simulink library "BrickPiSimSubLib_initreset"  (R2019a)
settings: Solver=VariableStepAuto  StartTime=0.0  StopTime=10.0  RelTol=1e-3
undefined symbols (not defined in the file or in its folder): A
libraries: BrickPiSimSubLib_Read x12, simulink x6, raspberrypilib x6
settings Model: Creator=hahn  LastModifiedBy=uk008555

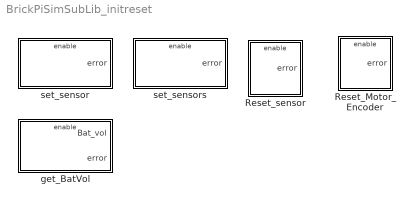
== system BrickPiSimSubLib_initreset ==
  Reset_Motor_Encoder : Subsystem  mask{Port_Val=A}
      mask prompts: Port_Val "Port"
      mask init:
      | switch Port_Val
      |     case 1
      |         d='A';
      |     case 2
      |         d='B';
      |     case 3
      |         d='C';
      |     otherwise
      |         d='D';
      | end
      mask TypeOptions Port_Val: Port_M/Port_Val
      mask Display: disp(['Reset\n Encoder \n Motor: ' d])
  Reset_sensor : Subsystem  mask{Port1_Val=on, Port2_Val=on, Port3_Val=on, Port4_Val=on}
      mask prompts: Port1_Val "Port1"; Port2_Val "Port2"; Port3_Val "Port3"; Port4_Val "Port4"
      mask init:
      | % d='';
      | % if Port1_Val
      | %     d=[d 'Sensor 1\n'];
      | % end
      | % if Port2_Val
      | %     d=[d 'Sensor 2\n'];
      | % end
      | % if Port3_Val
      | %     d=[d 'Sensor 3\n'];
      | % end
      | % if Port4_Val
      | %     d=[d 'Sensor 4'];
      | % end
      mask TypeOptions Port1_Val: Sensor_Ports/Port1_Val
      mask TypeOptions Port2_Val: Sensor_Ports/Port2_Val
      mask TypeOptions Port3_Val: Sensor_Ports/Port3_Val
      mask TypeOptions Port4_Val: Sensor_Ports/Port4_Val
      mask Display:
      | % disp(d)
      | [~,idx]=find([Port1_Val Port2_Val Port3_Val Port4_Val]);
      | disp(['Reset\n Sensor\n' num2str(idx)])
  get_BatVol : Subsystem
      mask Display: disp('Get\n VOLTAGE_BAT')
  set_sensor : Subsystem  mask{Type_Val=NXT Light on, Port_Val=3}
      mask prompts: Type_Val "Sensor Type:"; Port_Val "Port"
      mask init:
      | names = {
      |                   'NONE'
      |                   'I2C'
      |                   'CUSTOM'  % Choose 9v pullup, pin 5 and 6 configuration, and what to read back (ADC 1 and/or ADC 6 (always reports digital 5 and 6)).
      | 
      |                   'TOUCH'   % Touch sensor. When this mode is selected, automatically configure for NXT/EV3 as necessary.
      |                   'TOUCH_NXT' % 5
      |                   'TOUCH_EV3'
      | 
      |                   'NXT_LIGHT_ON'
      |                   'NXT_LIGHT_OFF'
      | 
      |                   'NXT_COLOR_RED'
      |                   'NXT_COLOR_GREEN'     % 10
      |                   'NXT_COLOR_BLUE'
      |                   'NXT_COLOR_FULL'
      |                   'NXT_COLOR_OFF'
      | 
      |                   'NXT_ULTRASONIC'
      | 
      |                   'EV3_GYRO_ABS'        % 15
      |                   'EV3_GYRO_DPS'
      |                   'EV3_GYRO_ABS_DPS'
      | 
      |                   'EV3_COLOR_REFLECTED'
      |                   'EV3_COLOR_AMBIENT'
      |                   'EV3_COLOR_COLOR'     % 20
      |                   'EV3_COLOR_RAW_REFLECTED'
      |                   'EV3_COLOR_COLOR_COMPONENTS'
      | 
      |                   'EV3_ULTRASONIC_CM'
      |                   'EV3_ULTRASONIC_INCHES'
      |                   'EV3_ULTRASONIC_LISTEN'   %25
      | 
      |                   'EV3_INFRARED_PROXIMITY'
      |                   'EV3_INFRARED_SEEK'
      |                   'EV3_INFRARED_REMOTE'};
      mask TypeOptions Type_Val: Sensor_Type/Type_Val
      mask TypeOptions Port_Val: Port_S/Port_Val
      mask Display:
      | % disp(['Address: ' num2str(Add_Val) '\n SensorTyp: ' num2str(Type_Val) '\n Port: ' num2str(Port_Val)])
      | disp(['Set \n' names{Type_Val} '\n Port: ' num2str(Port_Val)])
  set_sensors : Subsystem  mask{Type_Val=NXT Light on, Port1_Val=off, Port2_Val=on, Port3_Val=off, Port4_Val=on}
      mask prompts: Type_Val "Sensor Type:"; Port1_Val "Port1"; Port2_Val "Port2"; Port3_Val "Port3"; Port4_Val "Port4"
      mask init: same as BrickPiSimSubLib_initreset/set_sensor
      mask TypeOptions Type_Val: Sensor_Type/Type_Val
      mask TypeOptions Port1_Val: Sensor_Ports/Port1_Val
      mask TypeOptions Port2_Val: Sensor_Ports/Port2_Val
      mask TypeOptions Port3_Val: Sensor_Ports/Port3_Val
      mask TypeOptions Port4_Val: Sensor_Ports/Port4_Val
      mask Display:
      | [~,idx]=find([Port1_Val Port2_Val Port3_Val Port4_Val]);
      | disp(['Set\n'  names{Type_Val} '\n Port: ' num2str(idx)])
      | % num2str(Port1_Val+Port2_Val*2+Port3_Val*4+Port4_Val*8)

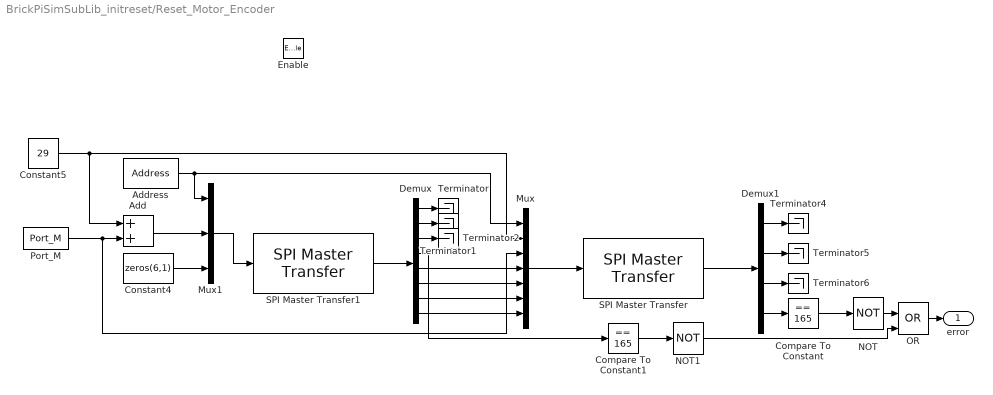
== system BrickPiSimSubLib_initreset/Reset_Motor_Encoder ==
  Enable : EnablePort
  Add : Sum
  Address : BrickPiSimSubLib_Read/Address  Add_Val=1
      settings: SourceProductName=Simulink Support Package for BrickPi
  Compare To Constant : simulink/Logic and Bit Operations/Compare To Constant  relop===  const=165  OutDataTypeStr=boolean
  Compare To Constant1 : simulink/Logic and Bit Operations/Compare To Constant  relop===  const=165  OutDataTypeStr=boolean
  Constant4 : Constant  Value=zeros(6,1)  OutDataTypeStr=uint8
  Constant5 : Constant  Value=29  OutDataTypeStr=uint8
  Demux : Demux  Outputs=8
  Demux1 : Demux
  Mux : Mux  Inputs=7
  Mux1 : Mux  Inputs=3
  NOT : Logic  Operator=NOT  IconShape=distinctive  AllPortsSameDT=off  OutDataTypeStr=boolean
  NOT1 : Logic  Operator=NOT  IconShape=distinctive  AllPortsSameDT=off  OutDataTypeStr=boolean
  OR : Logic  Operator=OR  IconShape=distinctive  AllPortsSameDT=off  OutDataTypeStr=boolean
  Port_M : BrickPiSimSubLib_Read/Port_M  Port_Val=A
      settings: SourceProductName=Simulink Support Package for BrickPi
  SPI Master Transfer : raspberrypilib/SPI Master Transfer  BoardProperty=Pi 3 Model B+  SPIModule=uint32(0)  Mode=Master  BusSpeed=1000000  Pin=SPI0_CE1  FirstBitToTransfer=Most significant bit (MSB)  ClockMode=0  BlockFunction=Transfer  RegisterAddress=0  OutputDataType=int8  OutputDataLength=1
      settings: SourceProductName=Simulink Support Package for Raspberry Pi Hardware  SourceProductBaseCode=RASPPI
  SPI Master Transfer1 : raspberrypilib/SPI Master Transfer  BoardProperty=Pi 3 Model B+  SPIModule=uint32(0)  Mode=Master  BusSpeed=1000000  Pin=SPI0_CE1  FirstBitToTransfer=Most significant bit (MSB)  ClockMode=0  BlockFunction=Transfer  RegisterAddress=0  OutputDataType=int8  OutputDataLength=1
      settings: SourceProductName=Simulink Support Package for Raspberry Pi Hardware  SourceProductBaseCode=RASPPI
  Terminator{,1..2,4..6} (6 alike) : Terminator
  error : Outport
  wires:
  Address/1 -> Mux1/1, Mux/1
  Mux/1 -> SPI Master Transfer/1
  Mux1/1 -> SPI Master Transfer1/1
  Add/1 -> Mux1/2
  Constant4/1 -> Mux1/3
  Constant5/1 -> Mux/2, Add/1
  Demux/8 -> Mux/7
  Demux/7 -> Mux/6
  Demux/6 -> Mux/5
  Demux/5 -> Mux/4
  SPI Master Transfer1/1 -> Demux/1
  Demux/1 -> Terminator/1
  Demux/2 -> Terminator1/1
  Demux/3 -> Terminator2/1
  Demux/4 -> Compare To Constant1/1
  Port_M/1 -> Mux/3, Add/2
  Demux1/3 -> Terminator6/1
  Compare To Constant/1 -> NOT/1
  Demux1/2 -> Terminator5/1
  Demux1/4 -> Compare To Constant/1
  Demux1/1 -> Terminator4/1
  SPI Master Transfer/1 -> Demux1/1
  Compare To Constant1/1 -> NOT1/1
  NOT1/1 -> OR/2
  NOT/1 -> OR/1
  OR/1 -> error/1

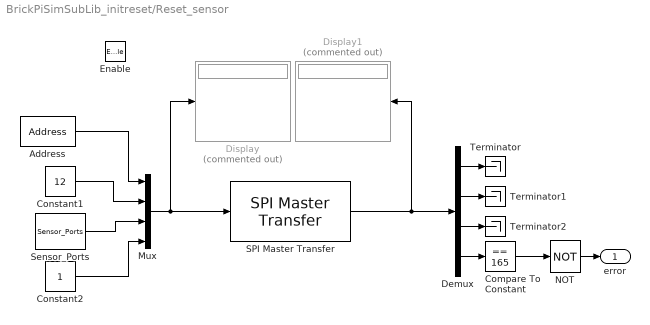
== system BrickPiSimSubLib_initreset/Reset_sensor ==
  Enable : EnablePort
  Address : BrickPiSimSubLib_Read/Address  Add_Val=1
      settings: SourceProductName=Simulink Support Package for BrickPi
  Compare To Constant : simulink/Logic and Bit Operations/Compare To Constant  relop===  const=165  OutDataTypeStr=boolean
  Constant1 : Constant  Value=12  OutDataTypeStr=uint8
  Constant2 : Constant  OutDataTypeStr=uint8
  Demux : Demux
  Display : Display  Commented=on
  Display1 : Display  Commented=on
  Mux : Mux
  NOT : Logic  Operator=NOT  IconShape=distinctive  AllPortsSameDT=off  OutDataTypeStr=boolean
  SPI Master Transfer : raspberrypilib/SPI Master Transfer  BoardProperty=Pi 3 Model B+  SPIModule=uint32(0)  Mode=Master  BusSpeed=1000000  Pin=SPI0_CE1  FirstBitToTransfer=Most significant bit (MSB)  ClockMode=0  BlockFunction=Transfer  RegisterAddress=0  OutputDataType=int8  OutputDataLength=1
      settings: SourceProductName=Simulink Support Package for Raspberry Pi Hardware  SourceProductBaseCode=RASPPI
  Sensor_Ports : BrickPiSimSubLib_Read/Sensor_Ports  Port1_Val=on  Port2_Val=on  Port3_Val=on  Port4_Val=on
      settings: SourceProductName=Simulink Support Package for BrickPi
  Terminator : Terminator
  Terminator1 : Terminator
  Terminator2 : Terminator
  error : Outport
  wires:
  Constant1/1 -> Mux/2
  Mux/1 -> Display/1, SPI Master Transfer/1
  Sensor_Ports/1 -> Mux/3
  Constant2/1 -> Mux/4
  Address/1 -> Mux/1
  NOT/1 -> error/1
  Compare To Constant/1 -> NOT/1
  Demux/3 -> Terminator2/1
  Demux/2 -> Terminator1/1
  Demux/1 -> Terminator/1
  Demux/4 -> Compare To Constant/1
  SPI Master Transfer/1 -> Demux/1, Display1/1

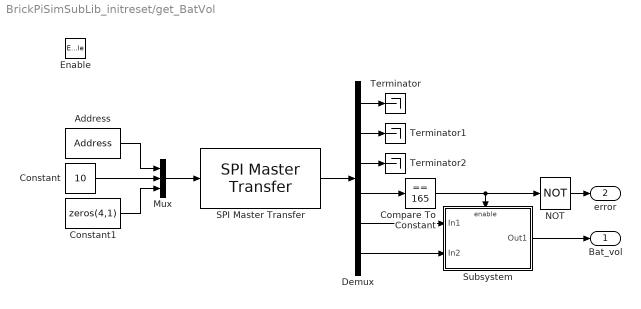
== system BrickPiSimSubLib_initreset/get_BatVol ==
  Enable : EnablePort
  Address : BrickPiSimSubLib_Read/Address  Add_Val=1
      settings: SourceProductName=Simulink Support Package for BrickPi
  Compare To Constant : simulink/Logic and Bit Operations/Compare To Constant  relop===  const=165  OutDataTypeStr=boolean
  Constant : Constant  Value=10  OutDataTypeStr=uint8
  Constant1 : Constant  Value=zeros(4,1)  OutDataTypeStr=uint8
  Demux : Demux  Outputs=6
  Mux : Mux  Inputs=3
  NOT : Logic  Operator=NOT  IconShape=distinctive  AllPortsSameDT=off  OutDataTypeStr=boolean
  SPI Master Transfer : raspberrypilib/SPI Master Transfer  BoardProperty=Pi 2 Model B  SPIModule=uint32(0)  Mode=Master  BusSpeed=1000000  Pin=SPI0_CE1  FirstBitToTransfer=Most significant bit (MSB)  ClockMode=0  BlockFunction=Transfer  RegisterAddress=0  OutputDataType=int8  OutputDataLength=1
      settings: SourceProductName=Simulink Support Package for Raspberry Pi Hardware  SourceProductBaseCode=RASPPI
  Subsystem : Subsystem
  Terminator : Terminator
  Terminator1 : Terminator
  Terminator2 : Terminator
  Bat_vol : Outport
  error : Outport  Port=2
  wires:
  Constant/1 -> Mux/2
  Constant1/1 -> Mux/3
  Address/1 -> Mux/1
  Mux/1 -> SPI Master Transfer/1
  SPI Master Transfer/1 -> Demux/1
  Demux/1 -> Terminator/1
  Demux/2 -> Terminator1/1
  Demux/3 -> Terminator2/1
  Demux/4 -> Compare To Constant/1
  Demux/5 -> Subsystem/1(In1)
  Demux/6 -> Subsystem/2(In2)
  Subsystem/1(Out1) -> Bat_vol/1
  Compare To Constant/1 -> NOT/1, Subsystem/Enable
  NOT/1 -> error/1

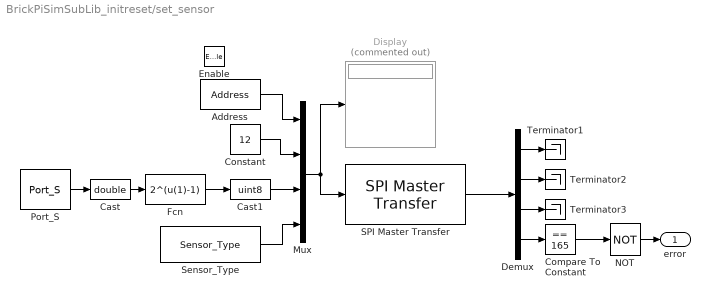
== system BrickPiSimSubLib_initreset/set_sensor ==
  Enable : EnablePort  StatesWhenEnabling=reset
  Address : BrickPiSimSubLib_Read/Address  Add_Val=1
      settings: SourceProductName=Simulink Support Package for BrickPi
  Cast : DataTypeConversion  OutDataTypeStr=double
  Cast1 : DataTypeConversion  OutDataTypeStr=uint8
  Compare To Constant : simulink/Logic and Bit Operations/Compare To Constant  relop===  const=165  OutDataTypeStr=boolean
  Constant : Constant  Value=12  OutDataTypeStr=uint8
  Demux : Demux
  Display : Display  Commented=on
  Fcn : Fcn  Expr=2^(u(1)-1)
  Mux : Mux
  NOT : Logic  Operator=NOT  IconShape=distinctive  AllPortsSameDT=off  OutDataTypeStr=boolean
  Port_S : BrickPiSimSubLib_Read/Port_S  Port_Val=3
      settings: SourceProductName=Simulink Support Package for BrickPi
  SPI Master Transfer : raspberrypilib/SPI Master Transfer  BoardProperty=Pi 3 Model B+  SPIModule=uint32(0)  Mode=Master  BusSpeed=1000000  Pin=SPI0_CE1  FirstBitToTransfer=Most significant bit (MSB)  ClockMode=0  BlockFunction=Transfer  RegisterAddress=0  OutputDataType=int8  OutputDataLength=1
      settings: SourceProductName=Simulink Support Package for Raspberry Pi Hardware  SourceProductBaseCode=RASPPI
  Sensor_Type : BrickPiSimSubLib_Read/Sensor_Type  Type_Val=NXT Light on
      settings: SourceProductName=Simulink Support Package for BrickPi
  Terminator1 : Terminator
  Terminator2 : Terminator
  Terminator3 : Terminator
  error : Outport
  wires:
  Mux/1 -> SPI Master Transfer/1, Display/1
  SPI Master Transfer/1 -> Demux/1
  Address/1 -> Mux/1
  Constant/1 -> Mux/2
  Sensor_Type/1 -> Mux/4
  Port_S/1 -> Cast/1
  Fcn/1 -> Cast1/1
  Cast/1 -> Fcn/1
  Cast1/1 -> Mux/3
  Demux/3 -> Terminator3/1
  Compare To Constant/1 -> NOT/1
  Demux/2 -> Terminator2/1
  Demux/4 -> Compare To Constant/1
  NOT/1 -> error/1
  Demux/1 -> Terminator1/1

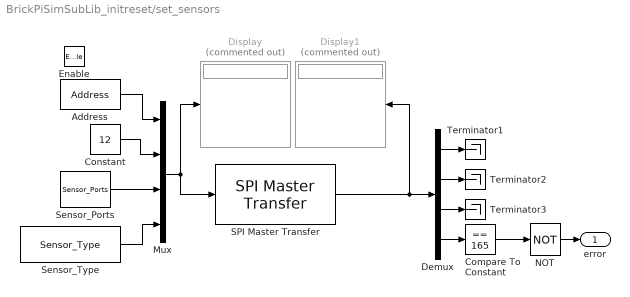
== system BrickPiSimSubLib_initreset/set_sensors ==
  Enable : EnablePort
  Address : BrickPiSimSubLib_Read/Address  Add_Val=1
      settings: SourceProductName=Simulink Support Package for BrickPi
  Compare To Constant : simulink/Logic and Bit Operations/Compare To Constant  relop===  const=165  OutDataTypeStr=boolean
  Constant : Constant  Value=12  OutDataTypeStr=uint8
  Demux : Demux
  Display : Display  Commented=on
  Display1 : Display  Commented=on
  Mux : Mux
  NOT : Logic  Operator=NOT  IconShape=distinctive  AllPortsSameDT=off  OutDataTypeStr=boolean
  SPI Master Transfer : raspberrypilib/SPI Master Transfer  BoardProperty=Pi 2 Model B  SPIModule=uint32(0)  Mode=Master  BusSpeed=1000000  Pin=SPI0_CE1  FirstBitToTransfer=Most significant bit (MSB)  ClockMode=0  BlockFunction=Transfer  RegisterAddress=0  OutputDataType=int8  OutputDataLength=1
      settings: SourceProductName=Simulink Support Package for Raspberry Pi Hardware  SourceProductBaseCode=RASPPI
  Sensor_Ports : BrickPiSimSubLib_Read/Sensor_Ports  Port1_Val=off  Port2_Val=on  Port3_Val=off  Port4_Val=on
      settings: SourceProductName=Simulink Support Package for BrickPi
  Sensor_Type : BrickPiSimSubLib_Read/Sensor_Type  Type_Val=NXT Light on
      settings: SourceProductName=Simulink Support Package for BrickPi
  Terminator1 : Terminator
  Terminator2 : Terminator
  Terminator3 : Terminator
  error : Outport
  wires:
  Sensor_Type/1 -> Mux/4
  Constant/1 -> Mux/2
  Address/1 -> Mux/1
  Mux/1 -> Display/1, SPI Master Transfer/1
  Sensor_Ports/1 -> Mux/3
  Demux/3 -> Terminator3/1
  Compare To Constant/1 -> NOT/1
  Demux/2 -> Terminator2/1
  Demux/4 -> Compare To Constant/1
  NOT/1 -> error/1
  Demux/1 -> Terminator1/1
  SPI Master Transfer/1 -> Demux/1, Display1/1

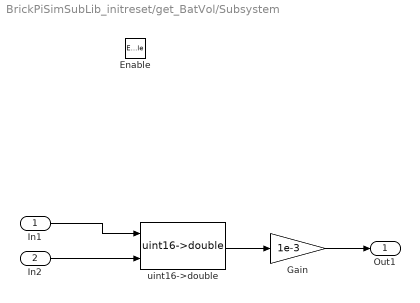
== system BrickPiSimSubLib_initreset/get_BatVol/Subsystem ==
  In1 : Inport
  In2 : Inport  Port=2
  Enable : EnablePort
  Gain : Gain  Gain=1e-3
  uint16->double : BrickPiSimSubLib_Read/uint16->double  SystemSampleTime=-1
      settings: SourceProductName=Simulink Support Package for BrickPi
  Out1 : Outport
  wires:
  In2/1 -> uint16->double/2
  In1/1 -> uint16->double/1
  uint16->double/1 -> Gain/1
  Gain/1 -> Out1/1
